simulink model "omega2thrust"  (Simulink 9.2)
settings: Solver=ode3  StartTime=0.0  StopTime=10.0  FixedStep=Ts  RelTol=1e-3  EnableMultiTasking=on
values from neighbouring files (symbols this model uses):
  b = 2e-09    [dataset.mat]    (also in initiateVars.m; system_workspace.mat; system_workspace_ayk.mat)
  k = 2.2e-08    [dataset.mat]    (also in initiateVars.m; system_workspace.mat; system_workspace_ayk.mat)
  l = 0.046    [dataset.mat]    (also in initiateVars.m; system_workspace.mat; system_workspace_ayk.mat)
settings Model: Creator=mgreiff  LastModifiedBy=aykut
settings DataIOCC: LimitDataPoints=off  SaveFormat=Dataset  SignalLoggingSaveFormat=Dataset
settings DebuggingCC: UnderspecifiedInitializationDetection=Simplified  MergeDetectMultiDrivingBlocksExec=error  FcnCallInpInsideContextMsg=error  StateNameClashWarn=none  SFExecutionAtInitializationDiag=warning
settings HardwareCC: ProdBitPerPointer=64  ProdBitPerSizeT=64  ProdBitPerPtrDiffT=64  ProdLargestAtomicFloat=Float  ProdIntDivRoundTo=Zero  ProdEndianess=LittleEndian  ProdWordSize=64  ProdHWDeviceType=Intel->x86-64 (Windows64)
settings ModelReferenceCC: PropagateSignalLabelsOutOfModel=on
settings GRTTargetCC: CombineOutputUpdateFcns=on  GRTInterface=off

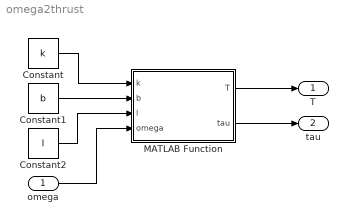
== system omega2thrust ==
  omega : Inport  PortDimensions=4
  Constant : Constant  Value=k
  Constant1 : Constant  Value=b
  Constant2 : Constant  Value=l
  MATLAB Function : MATLAB Function  TreatAsAtomicUnit=on
  T : Outport  PortDimensions=1
  tau : Outport  Port=2  PortDimensions=3
  wires:
  Constant/1 -> MATLAB Function/1(k)
  omega/1 -> MATLAB Function/4(omega)
  MATLAB Function/1(T) -> T/1
  Constant2/1 -> MATLAB Function/3(l)
  Constant1/1 -> MATLAB Function/2(b)
  MATLAB Function/2(tau) -> tau/1

== matlab function MATLAB Function ==
  data: k input double; b input double; l input double; T output double; omega input double; tau output double
function [T, tau]= fcn(k, b,l, omega)
%#codegen
omegasq = omega.^2;
Mw = [k   , k   , k  , k  ;
      0   , -k*l, 0  , k*l;
      -k*l, 0   , k*l, 0  ;
      -b  , b   , -b , b  ];
Tbar = Mw*omegasq;
T = Tbar(1);
tau = Tbar(2:4);
